simulink model "Rotorsimulation_Param_2019b"  (Simulink 10.0)
settings: Solver=ode3  StartTime=0.0  StopTime=1000  FixedStep=0.01  RelTol=1e-3  EnableMultiTasking=on
PostLoadFcn:
  | initRotorsimulation;
values from neighbouring files (symbols this model uses):
  BEMTPitchMax_deg = -30.0    [DD_Mdl.sldd]    (also in initRotorsimulationNREL5MW.m = -30)
  BladeLength_m = 61.5    [DD_Mdl.sldd]    (also in initRotorsimulationNREL5MW.m)
  BladeMass_kg = 17740.0    [DD_Mdl.sldd]    (also in initRotorsimulationNREL5MW.m = 17740)
  BladePitchMax_deg = 0.0    [DD_Mdl.sldd]    (also in initRotorsimulationNREL5MW.m = 0)
  BladePitchrateNorm_degpers = 3.0    [DD_Mdl.sldd]    (also in initRotorsimulationNREL5MW.m = 3)
  BladePitchrateStop_degpers = 9.0    [DD_Mdl.sldd]    (also in initRotorsimulationNREL5MW.m = 9)
  BladePitchStart_deg = -85.0    [DD_Mdl.sldd]    (also in initRotorsimulationNREL5MW.m = -85)
  BladePrecone_deg = 2.5    [DD_Mdl.sldd]    (also in initRotorsimulationNREL5MW.m)
  BladeTwist_deg = 13.308 13.308 13.308 13.308 13.308 13.308 13.308 13.308 13.308 13.308 13.308 13.308 13.181 12.848 12.192 11.561 11.072 10.792 10.232 9.672 9.11 8.534 7.932 7.321 6.711 6.122 5.546 4.971 4.401 3.834 3.332 2.89 2.503 2.116 1.73 1.342 0.954 0.76 0.574 0.404 0.319 0.253 0.216 0.178 0.14 0.101 0.062 0.023 0.0    [DD_Mdl.sldd]    (also in initRotorsimulationNREL5MW.m = [13.308 13.308 13.308 13.308 13.308 13.308 13.308 13.308 13.)
  cperR = 0.054 0.054 0.056 0.058 0.06 0.061 0.063 0.065 0.067 0.069 0.07 0.072 0.073 0.073 0.073 0.074 0.073 0.072 0.071 0.069 0.068 0.066 0.064 0.062 0.06 0.058 0.056 0.054 0.052 0.05 0.049 0.047 0.045 0.043 0.041 0.039 0.037 0.036 0.035 0.033 0.032 0.03 0.028 0.026 0.024 0.022 0.02 0.018 0.017    [DD_Mdl.sldd]    (also in initRotorsimulationNREL5MW.m = [0.054 0.054 0.056 0.058 0.060 0.061 0.063 0.065 0.067 0.069)
  Cut_OffWindSpeed_mpers = 25.0    [DD_Mdl.sldd]    (also in initRotorsimulationNREL5MW.m = 25)
  DownwashCorrection = 0.26    [DD_Mdl.sldd]    (also in initRotorsimulationNREL5MW.m)
  DownwashModelSwitch = 3.0    [DD_Mdl.sldd]    (also in initRotorsimulationNREL5MW.m = 3)
  drperR = 0.024 0.003 0.016 0.016 0.016 0.016 0.016 0.016 0.016 0.016 0.016 0.016 0.016 0.016 0.016 0.016 0.016 0.016 0.032 0.032 0.032 0.032 0.032 0.032 0.032 0.032 0.032 0.032 0.032 0.032 0.032 0.032 0.032 0.032 0.032 0.032 0.032 0.016 0.016 0.016 0.008 0.008 0.008 0.008 0.008 0.008 0.008 0.008 0.005    [DD_Mdl.sldd]    (also in initRotorsimulationNREL5MW.m = [0.024 0.003 0.016 0.016 0.016 0.016 0.016 0.016 0.016 0.016)
  DT_s = 0.008    [DD_Mdl.sldd]    (also in initRotorsimulationNREL5MW.m = 0.01)
  g_mpers_2 = 9.81    [DD_Mdl.sldd]    (also in initRotorsimulationNREL5MW.m)
  GeneratorEfficiency = 0.944    [DD_Mdl.sldd]    (also in initRotorsimulationNREL5MW.m)
  GeneratorOptimalModeGain_Nmper_radpers2 = 2128600    [initRotorsimulationNREL5MW.m]
  HubRadius_m = 1.5    [DD_Mdl.sldd]    (also in initRotorsimulationNREL5MW.m)
  Ki = 0.3    [initRotorsimulationNREL5MW.m]
  Kp = 0.1    [initRotorsimulationNREL5MW.m]
  mpermBl = 0.058 0.008 0.044 0.043 0.042 0.034 0.026 0.024 0.023 0.022 0.023 0.024 0.024 0.023 0.022 0.02 0.02 0.02 0.039 0.038 0.037 0.036 0.034 0.033 0.03 0.029 0.028 0.025 0.023 0.021 0.019 0.018 0.016 0.015 0.012 0.011 0.01 0.005 0.004 0.004 0.002 0.002 0.002 0.002 0.001 0.001 0.001 0.0 0.0    [DD_Mdl.sldd]    (also in initRotorsimulationNREL5MW.m = [0.058 0.008 0.044 0.043 0.042 0.034 0.026 0.024 0.023 0.022)
  nBl = 3.0    [DD_Mdl.sldd]    (also in initRotorsimulationNREL5MW.m = 3)
  nR = 49.0    [DD_Mdl.sldd]    (also in initRotorsimulationNREL5MW.m = length(drperR))
  Overhang_m = 5.0    [DD_Mdl.sldd]    (also in initRotorsimulationNREL5MW.m = 5)
  RatedOmega_RPM = 12.1    [DD_Mdl.sldd]    (also in initRotorsimulationNREL5MW.m)
  RatedWindSpeed_mpers = 11.4    [DD_Mdl.sldd]    (also in initRotorsimulationNREL5MW.m)
  rho_kgperm3 = 1.225    [DD_Mdl.sldd]    (also in initRotorsimulationNREL5MW.m)
  rperR = 0.024 0.027 0.043 0.059 0.075 0.09 0.106 0.122 0.138 0.154 0.17 0.186 0.202 0.217 0.233 0.249 0.265 0.281 0.313 0.344 0.376 0.408 0.44 0.471 0.503 0.535 0.567 0.598 0.63 0.662 0.694 0.725 0.757 0.789 0.821 0.852 0.884 0.9 0.916 0.932 0.94 0.948 0.956 0.963 0.971 0.979 0.987 0.995 1.0    [DD_Mdl.sldd]    (also in initRotorsimulationNREL5MW.m = [0.024 0.027 0.043 0.059 0.075 0.090 0.106 0.122 0.138 0.154)
  Shafttilt_deg = 5.0    [DD_Mdl.sldd]    (also in initRotorsimulationNREL5MW.m = 5)
  TipSpeedLoss = 0.0    [DD_Mdl.sldd]    (also in initRotorsimulationNREL5MW.m = 0)
  TowerDamOnperoff = 0.0    [DD_Mdl.sldd]    (also in initRotorsimulationNREL5MW.m = 0)
  TowerDragCoefficient = 0.35    [DD_Mdl.sldd]    (also in initRotorsimulationNREL5MW.m)
  TowerRadius_m = 1.935    [DD_Mdl.sldd]    (also in initRotorsimulationNREL5MW.m)
libraries: simulink x7
(part 1 of 2)
settings Model: Creator=rbartels  LastModifiedBy=ditt_aj
settings DataIOCC: LimitDataPoints=on  SignalLoggingSaveFormat=ModelDataLogs
settings OptimizationCC: ExpressionDepthLimit=2147483647  InitFltsAndDblsToZero=on
settings DebuggingCC: SolverPrmCheckMsg=warning  FcnCallInpInsideContextMsg=warning  StateNameClashWarn=warning
settings SFSimCC: SimUseLocalCustomCode=on
settings RTWCC: RTWUseLocalCustomCode=on

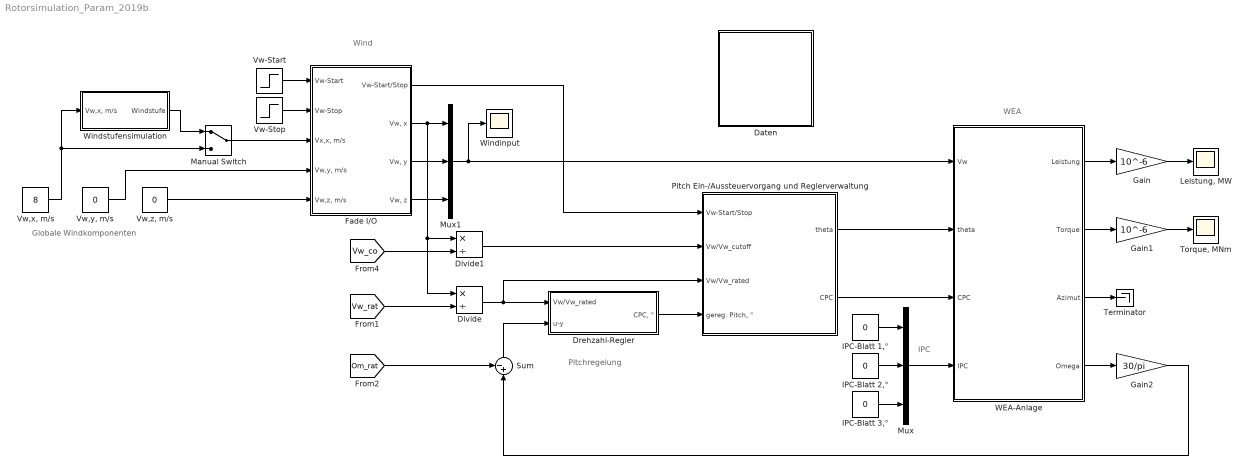
== system Rotorsimulation_Param_2019b ==
  note: Wind
  note: Pitchregelung
  note: IPC
  note: WEA
  note: Globale Windkomponenten
  Daten : Subsystem
  Divide : Product  Inputs=*/
  Divide1 : Product  Inputs=*/
  Drehzahl-Regler : Subsystem
  Fade I/O : Subsystem
  Gain : Gain  Gain=10^-6
  Gain1 : Gain  Gain=10^-6
  Gain2 : Gain  Gain=30/pi
  IPC-Blatt 1,° : Constant  Value=0
  IPC-Blatt 2,° : Constant  Value=0
  IPC-Blatt 3,° : Constant  Value=0
  "Leistung, MW" : Scope
  Manual Switch : ManualSwitch
  Mux : Mux  Inputs=3
  Mux1 : Mux  Inputs=3
  Pitch Ein-/Aussteuervorgang und Reglerverwaltung : Subsystem
  Sum : Sum  Inputs=-+|
  Terminator : Terminator
  "Torque, MNm" : Scope
  "Vw,x, m/s " : Constant  Value=8
  "Vw,y, m/s" : Constant  Value=0
  "Vw,z, m/s" : Constant  Value=0
  Vw-Start : Step  SampleTime=0
  Vw-Stop : Step  Time=2000  Before=1  After=0  SampleTime=0
  WEA-Anlage : Subsystem
  Windinput : Scope
  Windstufensimulation : Subsystem
  wires:
  Fade I/O/2("Vw, x") -> Mux1/1, Divide/1, Divide1/1
  Vw-Start/1 -> Fade I/O/1(Vw-Start)
  Vw-Stop/1 -> Fade I/O/2(Vw-Stop)
  WEA-Anlage/1(Leistung) -> Gain/1
  "Vw,y, m/s"/1 -> Fade I/O/4("Vw,y, m/s")
  "Vw,z, m/s"/1 -> Fade I/O/5("Vw,z, m/s")
  Fade I/O/4("Vw, z") -> Mux1/3
  Fade I/O/3("Vw, y") -> Mux1/2
  WEA-Anlage/2(Torque) -> Gain1/1
  Gain/1 -> "Leistung, MW"/1
  Gain1/1 -> "Torque, MNm"/1
  IPC-Blatt 3,°/1 -> Mux/3
  WEA-Anlage/3(Azimut) -> Terminator/1
  WEA-Anlage/4(Omega) -> Gain2/1
  Sum/1 -> Drehzahl-Regler/2(u-y)
  Drehzahl-Regler/1("CPC, °") -> Pitch Ein-/Aussteuervorgang und Reglerverwaltung/4("gereg. Pitch, °")
  [Vw_rat] -> Divide/2
  Divide/1 -> Drehzahl-Regler/1(Vw/Vw_rated), Pitch Ein-/Aussteuervorgang und Reglerverwaltung/3(Vw/Vw_rated)
  [Om_rat] -> Sum/1
  Gain2/1 -> Sum/2
  Mux1/1 -> WEA-Anlage/1(Vw), Windinput/1
  Fade I/O/1(Vw-Start/Stop) -> Pitch Ein-/Aussteuervorgang und Reglerverwaltung/1(Vw-Start/Stop)
  Manual Switch/1 -> Fade I/O/3("Vx,x, m/s")
  "Vw,x, m/s "/1 -> Windstufensimulation/1("Vw,x, m/s"), Manual Switch/2
  Windstufensimulation/1(" Windstufe") -> Manual Switch/1
  Divide1/1 -> Pitch Ein-/Aussteuervorgang und Reglerverwaltung/2(Vw/Vw_cutoff)
  [Vw_co] -> Divide1/2
  IPC-Blatt 2,°/1 -> Mux/2
  IPC-Blatt 1,°/1 -> Mux/1
  Mux/1 -> WEA-Anlage/4(IPC)
  Pitch Ein-/Aussteuervorgang und Reglerverwaltung/2(CPC) -> WEA-Anlage/3(CPC)
  Pitch Ein-/Aussteuervorgang und Reglerverwaltung/1(theta) -> WEA-Anlage/2(theta)

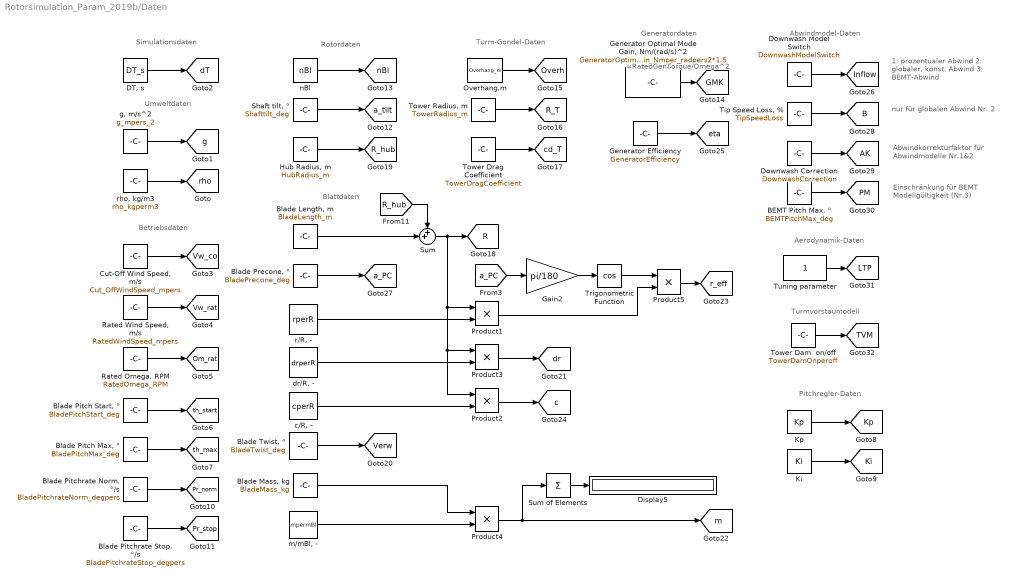
== system Rotorsimulation_Param_2019b/Daten ==
  note: Simulationsdaten
  note: Umweltdaten
  note: Betriebsdaten
  note: Pitchregler-Daten
  note: =RatedGenTorque/Omega^2
  note: Rotordaten
  note: Turm-Gondel-Daten
  note: Generatordaten
  note: Blattdaten
  note: 1: prozentualer Abwind
      | 2: globaler, konst. Abwind
      | 3: BEMT-Abwind
  note: Abwindmodel-Daten
  note: nur für globalen Abwind Nr. 2
  note: Abwindkorrekturfaktor für
      | Abwindmodelle Nr.1&2
  note: Einschränkung für BEMT
      | Modellgültigkeit (Nr.3)
  note: Aerodynamik-Daten
  note: Turmvorstaumodell
  "BEMT Pitch Max, °" : Constant  Value=BEMTPitchMax_deg
  "Blade Length, m" : Constant  Value=BladeLength_m
  "Blade Mass, kg" : Constant  Value=BladeMass_kg
  "Blade Pitch Max, °" : Constant  Value=BladePitchMax_deg
  "Blade Pitch Start, °" : Constant  Value=BladePitchStart_deg
  Blade Pitchrate Norm. °/s : Constant  Value=BladePitchrateNorm_degpers
  Blade Pitchrate Stop. °/s : Constant  Value=BladePitchrateStop_degpers
  "Blade Precone, °" : Constant  Value=BladePrecone_deg
  "Blade Twist, °" : Constant  Value=BladeTwist_deg
  "Cut-Off Wind Speed, m/s" : Constant  Value=Cut_OffWindSpeed_mpers
  "DT, s" : Constant  Value=DT_s
  Display5 : Display
  Downwash Correction : Constant  Value=DownwashCorrection
  Downwash Model Switch : Constant  Value=DownwashModelSwitch
  Gain2 : Gain  Gain=pi/180
  Generator Efficiency : Constant  Value=GeneratorEfficiency
  "Generator Optimal Mode Gain, Nm/(rad/s)^2" : Constant  Value=GeneratorOptimalModeGain_Nmper_radpers2*1.5
  "Hub Radius, m" : Constant  Value=HubRadius_m
  Ki : Constant  Value=Ki
  Kp : Constant  Value=Kp
  Overhang,m : Constant  Value=Overhang_m
  Product{1..5} (5 alike) : Product  RndMeth=Zero
  "Rated Omega, RPM" : Constant  Value=RatedOmega_RPM
  "Rated Wind Speed, m/s" : Constant  Value=RatedWindSpeed_mpers
  "Shaft tilt, °" : Constant  Value=Shafttilt_deg
  Sum : Sum  Inputs=++|
  Sum of Elements : Sum  Inputs=+
  "Tip Speed Loss, %" : Constant  Value=TipSpeedLoss
  Tower Dam  on/off : Constant  Value=TowerDamOnperoff
  Tower Drag Coefficient : Constant  Value=TowerDragCoefficient
  "Tower Radius, m" : Constant  Value=TowerRadius_m
  Trigonometric Function : Trigonometry  Operator=cos
  Tuning parameter : Constant
  "c/R, -" : Constant  Value=cperR
  "dr/R, -" : Constant  Value=drperR
  "g, m/s^2" : Constant  Value=g_mpers_2
  "m/mBl, - " : Constant  Value=mpermBl
  nBl : Constant  Value=nBl
  "r/R, -" : Constant  Value=rperR
  "rho, kg/m3" : Constant  Value=rho_kgperm3
  tag scope: AK=global, B=global, GMK=global, Inflow=global, Ki=global, Kp=global, LTP=global, Om_rat=global, Overh=global, PM=global, Pr_norm=global, Pr_stop=global, R=global, R_T=global, R_hub=global, TVM=global, Verw=global, Vw_co=global, Vw_rat=global, a_PC=global, a_tilt=global, c=global, cd_T=global, dT=global, dr=global, eta=global, g=global, m=global, nBl=global, r_eff=global, rho=global, th_max=global, th_start=global
  wires:
  "rho, kg/m3"/1 -> [rho]
  "g, m/s^2"/1 -> [g]
  "DT, s"/1 -> [dT]
  "Cut-Off Wind Speed, m/s"/1 -> [Vw_co]
  "Rated Wind Speed, m/s"/1 -> [Vw_rat]
  "Rated Omega, RPM"/1 -> [Om_rat]
  "Blade Pitch Start, °"/1 -> [th_start]
  "Blade Pitch Max, °"/1 -> [th_max]
  Ki/1 -> [Ki]
  Kp/1 -> [Kp]
  Blade Pitchrate Norm. °/s/1 -> [Pr_norm]
  Blade Pitchrate Stop. °/s/1 -> [Pr_stop]
  nBl/1 -> [nBl]
  "Generator Optimal Mode Gain, Nm/(rad/s)^2"/1 -> [GMK]
  "Shaft tilt, °"/1 -> [a_tilt]
  Overhang,m/1 -> [Overh]
  "Tower Radius, m"/1 -> [R_T]
  Tower Drag Coefficient/1 -> [cd_T]
  "r/R, -"/1 -> Product1/2
  "c/R, -"/1 -> Product2/2
  "Blade Twist, °"/1 -> [Verw]
  "m/mBl, - "/1 -> Product4/2
  "dr/R, -"/1 -> Product3/2
  Sum of Elements/1 -> Display5/1
  Gain2/1 -> Trigonometric Function/1
  Trigonometric Function/1 -> Product5/1
  Product5/1 -> [r_eff]
  Product1/1 -> Product5/2
  Product3/1 -> [dr]
  Product2/1 -> [c]
  Product4/1 -> [m], Sum of Elements/1
  "Hub Radius, m"/1 -> [R_hub]
  Sum/1 -> [R], Product1/1, Product3/1, Product2/1
  "Blade Length, m"/1 -> Sum/2
  [R_hub] -> Sum/1
  "Blade Mass, kg"/1 -> Product4/1
  "Blade Precone, °"/1 -> [a_PC]
  [a_PC] -> Gain2/1
  Generator Efficiency/1 -> [eta]
  Downwash Model Switch/1 -> [Inflow]
  "Tip Speed Loss, %"/1 -> [B]
  Downwash Correction/1 -> [AK]
  "BEMT Pitch Max, °"/1 -> [PM]
  Tuning parameter/1 -> [LTP]
  Tower Dam  on/off/1 -> [TVM]

== system Rotorsimulation_Param_2019b/Drehzahl-Regler ==
  Vw/Vw_rated : Inport
  u-y : Inport  Port=2
  Diff : Constant  Value=0
  Gain3 : Gain  Gain=180/pi
  PI-Regler : Subsystem
  Saturation Dynamic : simulink/Discontinuities/Saturation Dynamic  OutMin=[]  OutMax=[]  OutDataTypeStr=Inherit: Same as second input  OutDataType=sfix(16)  OutScaling=2^-10  DoSatur=off
  Switch : Switch  Criteria=u2 > Threshold  Threshold=1
  Verstärkungen : Subsystem
  "CPC, °" : Outport  VectorParamsAs1DForOutWhenUnconnected=off
  wires:
  PI-Regler/1(e) -> Gain3/1
  Verstärkungen/1(Verstärkungen) -> PI-Regler/2(Verstärkungen)
  Gain3/1 -> Saturation Dynamic/2
  Saturation Dynamic/1 -> "CPC, °"/1
  [th_max] -> Saturation Dynamic/1
  [th_start] -> Saturation Dynamic/3
  Diff/1 -> Switch/3
  u-y/1 -> Switch/1  "diff"
  Vw/Vw_rated/1 -> Switch/2
  Switch/1 -> PI-Regler/1(u-y)

== system Rotorsimulation_Param_2019b/Fade I/O ==
  Vw-Start : Inport
  Vw-Stop : Inport  Port=2
  "Vx,x, m/s" : Inport  Port=3
  "Vw,y, m/s" : Inport  Port=4
  "Vw,z, m/s" : Inport  Port=5
  Demux : Demux  Outputs=3
  Mux2 : Mux  Inputs=3
  Product : Product  RndMeth=Zero
  Product1 : Product  RndMeth=Zero
  Rate Limiter1 : RateLimiter  SampleTimeMode=inherited
  Vw-Start/Stop : Outport  VectorParamsAs1DForOutWhenUnconnected=off
  "Vw, x" : Outport  Port=2  VectorParamsAs1DForOutWhenUnconnected=off
  "Vw, y" : Outport  Port=3  VectorParamsAs1DForOutWhenUnconnected=off
  "Vw, z" : Outport  Port=4  VectorParamsAs1DForOutWhenUnconnected=off
  tag scope: Vw_in=global
  wires:
  Product1/1 -> Rate Limiter1/1
  Rate Limiter1/1 -> Demux/1
  "Vx,x, m/s"/1 -> Mux2/1
  "Vw,y, m/s"/1 -> Mux2/2
  "Vw,z, m/s"/1 -> Mux2/3
  Mux2/1 -> Product1/2
  Demux/1 -> "Vw, x"/1, [Vw_in]
  Demux/3 -> "Vw, z"/1
  Demux/2 -> "Vw, y"/1
  Vw-Start/1 -> Product/1
  Vw-Stop/1 -> Product/2
  Product/1 -> Product1/1, Vw-Start/Stop/1

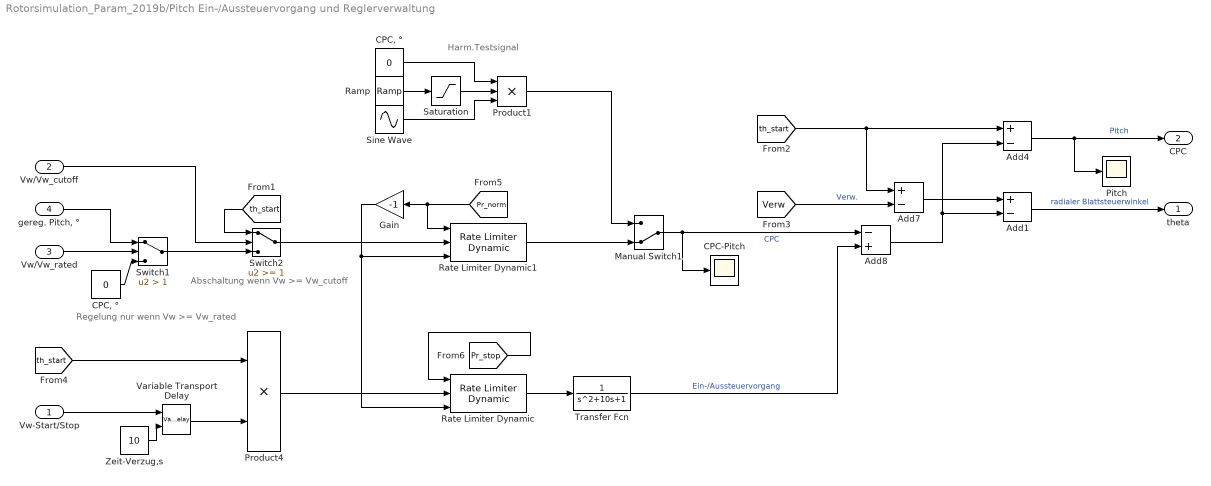
== system Rotorsimulation_Param_2019b/Pitch Ein-/Aussteuervorgang und Reglerverwaltung ==
  note: Harm.Testsignal
  note: Regelung nur wenn Vw >= Vw_rated
  note: Abschaltung wenn Vw >= Vw_cutoff
  Vw-Start/Stop : Inport
  Vw/Vw_cutoff : Inport  Port=2
  Vw/Vw_rated : Inport  Port=3
  "gereg. Pitch, °" : Inport  Port=4
  " CPC, ° " : Constant  Value=0
  " Pitch " : Scope
  Add1 : Sum  Inputs=+-
  Add4 : Sum  Inputs=+-
  Add7 : Sum  Inputs=+-
  Add8 : Sum  Inputs=-+
  "CPC, °" : Constant  Value=0
  CPC-Pitch : Scope
  Gain : Gain  Gain=-1
  Manual Switch1 : ManualSwitch  CurrentSetting=0
  Product1 : Product  Inputs=3  RndMeth=Zero
  Product4 : Product  RndMeth=Zero
  Ramp : simulink/Sources/Ramp  slope=0.1  start=200  InitialOutput=0
  Rate Limiter Dynamic : simulink/Discontinuities/Rate Limiter Dynamic
      settings: SourceProductName=Simulink
  Rate Limiter Dynamic1 : simulink/Discontinuities/Rate Limiter Dynamic
      settings: SourceProductName=Simulink
  Saturation : Saturate  UpperLimit=1  LowerLimit=0
  Sine Wave : Sin  Frequency=0.1  SampleTime=0
  Switch1 : Switch  Criteria=u2 > Threshold  Threshold=1
  Switch2 : Switch  Threshold=1
  Transfer Fcn : TransferFcn  Denominator=[1 10 1]
  Variable Transport Delay : VariableTransportDelay  VariableDelayType=Variable transport delay  MaximumDelay=10
  Zeit-Verzug,s : Constant  Value=10
  theta : Outport  VectorParamsAs1DForOutWhenUnconnected=off
  CPC : Outport  Port=2  VectorParamsAs1DForOutWhenUnconnected=off
  wires:
  Rate Limiter Dynamic/1 -> Transfer Fcn/1
  Product4/1 -> Rate Limiter Dynamic/2
  [th_start] -> Product4/1
  Transfer Fcn/1 -> Add8/2  "Ein-/Aussteuervorgang"
  Variable Transport Delay/1 -> Product4/2
  Vw-Start/Stop/1 -> Variable Transport Delay/1
  Zeit-Verzug,s/1 -> Variable Transport Delay/2
  [Pr_stop] -> Rate Limiter Dynamic/1
  Ramp/1 -> Saturation/1
  Sine Wave/1 -> Product1/3
  Saturation/1 -> Product1/2
  Product1/1 -> Manual Switch1/1
  " CPC, ° "/1 -> Switch1/3
  "CPC, °"/1 -> Product1/1
  Manual Switch1/1 -> Add8/1, CPC-Pitch/1  "CPC"
  Switch1/1 -> Switch2/3
  Switch2/1 -> Rate Limiter Dynamic1/2
  [th_start] -> Switch2/1
  Vw/Vw_cutoff/1 -> Switch2/2
  Vw/Vw_rated/1 -> Switch1/2
  "gereg. Pitch, °"/1 -> Switch1/1
  [th_start] -> Add4/1, Add7/1
  Add7/1 -> Add1/1
  [Verw] -> Add7/2  "Verw."
  Add4/1 -> " Pitch "/1, CPC/1  "Pitch"
  Add8/1 -> Add4/2, Add1/2
  Add1/1 -> theta/1  "radialer Blattsteuerwinkel"
  Rate Limiter Dynamic1/1 -> Manual Switch1/2
  [Pr_norm] -> Rate Limiter Dynamic1/1, Gain/1
  Gain/1 -> Rate Limiter Dynamic1/3, Rate Limiter Dynamic/3

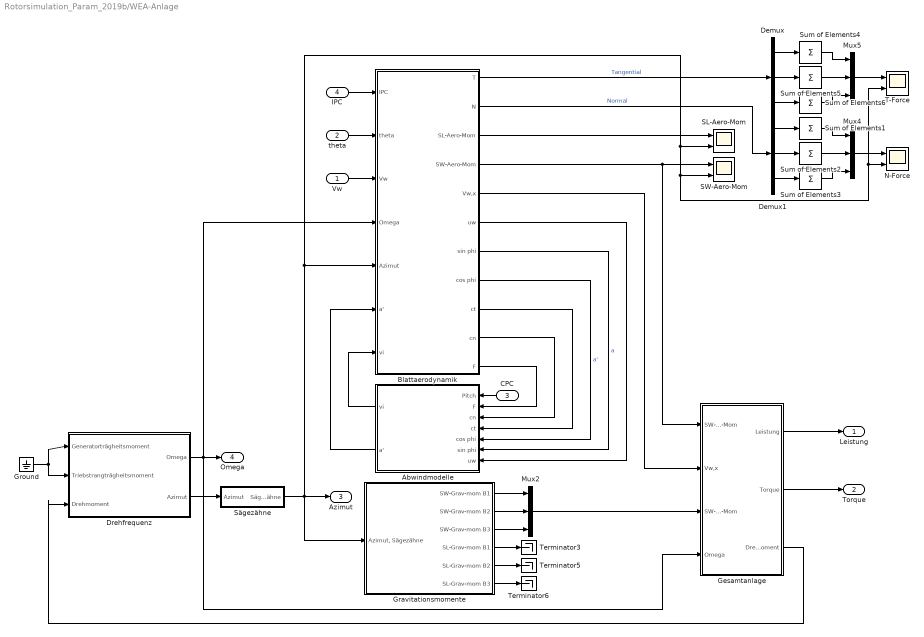
== system Rotorsimulation_Param_2019b/WEA-Anlage ==
  Vw : Inport
  theta : Inport  Port=2
  CPC : Inport  Port=3
  IPC : Inport  Port=4
  Abwindmodelle : Subsystem
  Blattaerodynamik : Subsystem
  Demux : Demux  Outputs=3
  Demux1 : Demux  Outputs=3
  Drehfrequenz : Subsystem
  Gesamtanlage : Subsystem
  Gravitationsmomente : Subsystem
  Ground : Ground
  Mux2 : Mux  Inputs=3
  Mux4 : Mux  Inputs=3
  Mux5 : Mux  Inputs=3
  N-Force : Scope  NumInputPorts=2
  SL-Aero-Mom : Scope  NumInputPorts=2
  SW-Aero-Mom : Scope  NumInputPorts=2
  Sum of Elements{1..6} (6 alike) : Sum  Inputs=+
  Sägezähne : Subsystem
  T-Force : Scope  NumInputPorts=2
  Terminator3 : Terminator
  Terminator5 : Terminator
  Terminator6 : Terminator
  Leistung : Outport  VectorParamsAs1DForOutWhenUnconnected=off
  Torque : Outport  Port=2  VectorParamsAs1DForOutWhenUnconnected=off
  Azimut : Outport  Port=3  VectorParamsAs1DForOutWhenUnconnected=off
  Omega : Outport  Port=4  VectorParamsAs1DForOutWhenUnconnected=off
  wires:
  Blattaerodynamik/1(T) -> Demux/1  "Tangential"
  Blattaerodynamik/2(N) -> Demux1/1  "Normal"
  Sägezähne/1(Sägezähne) -> Gravitationsmomente/1("Azimut, Sägezähne"), Blattaerodynamik/5(Azimut), SL-Aero-Mom/2, SW-Aero-Mom/2, N-Force/2, T-Force/2, Azimut/1
  Drehfrequenz/2(Azimut) -> Sägezähne/1(Azimut)
  Blattaerodynamik/4(SW-Aero-Mom) -> Gesamtanlage/1(SW-Aero-Mom), SW-Aero-Mom/1
  Blattaerodynamik/3(SL-Aero-Mom) -> SL-Aero-Mom/1
  Gravitationsmomente/1(SW-Grav-mom B1) -> Mux2/1
  Gravitationsmomente/2(SW-Grav-mom B2) -> Mux2/2
  Gravitationsmomente/3(SW-Grav-mom B3) -> Mux2/3
  Gesamtanlage/2(Torque) -> Torque/1
  Abwindmodelle/1(vi) -> Blattaerodynamik/7(vi)
  Blattaerodynamik/8(cos phi) -> Abwindmodelle/5(cos phi)  "a'"
  Blattaerodynamik/7(sin phi) -> Abwindmodelle/6(sin phi)  "a"
  Blattaerodynamik/10(cn) -> Abwindmodelle/3(cn)
  Blattaerodynamik/9(ct) -> Abwindmodelle/4(ct)
  Abwindmodelle/2(a') -> Blattaerodynamik/6(a')
  theta/1 -> Blattaerodynamik/2(theta)
  Blattaerodynamik/11(F) -> Abwindmodelle/2(F)
  Gravitationsmomente/4(SL-Grav-mom B1) -> Terminator3/1
  Gravitationsmomente/6(SL-Grav-mom B3) -> Terminator6/1
  Gravitationsmomente/5(SL-Grav-mom B2) -> Terminator5/1
  Vw/1 -> Blattaerodynamik/3(Vw)
  Drehfrequenz/1(Omega) -> Gesamtanlage/4(Omega), Omega/1, Blattaerodynamik/4(Omega)
  Mux2/1 -> Gesamtanlage/3(SW-Grav-Mom)
  Gesamtanlage/1(Leistung) -> Leistung/1
  Gesamtanlage/3(Drehmoment) -> Drehfrequenz/3(Drehmoment)
  Demux1/1 -> Sum of Elements1/1
  Demux1/2 -> Sum of Elements2/1
  Demux1/3 -> Sum of Elements3/1
  Sum of Elements1/1 -> Mux4/1
  Sum of Elements2/1 -> Mux4/2
  Mux4/1 -> N-Force/1
  Demux/1 -> Sum of Elements4/1
  Demux/2 -> Sum of Elements5/1
  Demux/3 -> Sum of Elements6/1
  Sum of Elements4/1 -> Mux5/1
  Sum of Elements6/1 -> Mux5/3
  Sum of Elements5/1 -> Mux5/2
  Mux5/1 -> T-Force/1
  Blattaerodynamik/5(Vw,x) -> Gesamtanlage/2(Vw,x)
  Blattaerodynamik/6(" uw") -> Abwindmodelle/7(uw)
  IPC/1 -> Blattaerodynamik/1(IPC)
  CPC/1 -> Abwindmodelle/1(Pitch)
  Ground/1 -> Drehfrequenz/1(Generatorträgheitsmoment), Drehfrequenz/2(Triebstrangträgheitsmoment)
  Sum of Elements3/1 -> Mux4/3

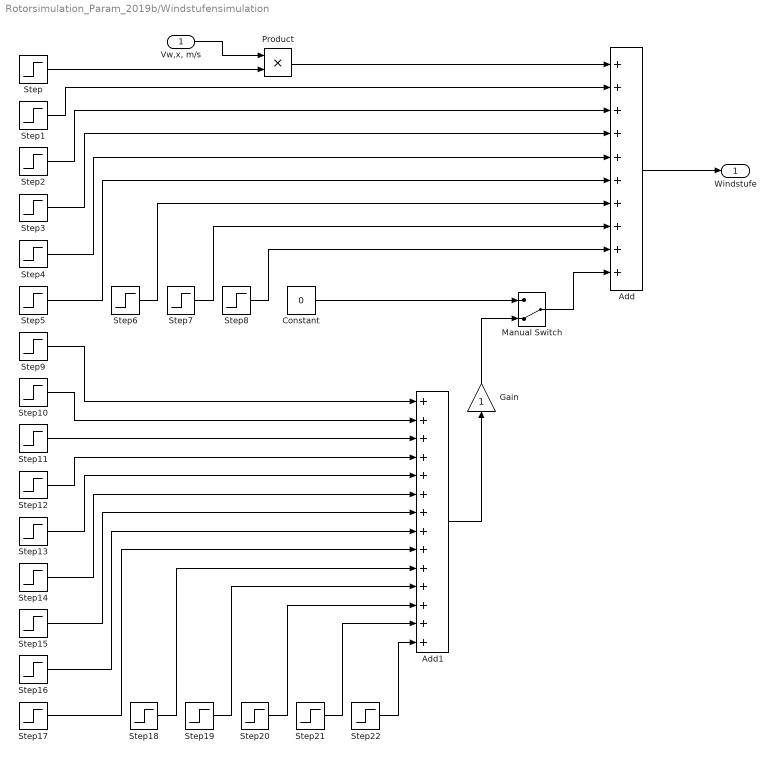
== system Rotorsimulation_Param_2019b/Windstufensimulation ==
  "Vw,x, m/s" : Inport
  Add : Sum  Inputs=++++++++++
  Add1 : Sum  Inputs=++++++++++++++
  Constant : Constant  Value=0
  Gain : Gain
  Manual Switch : ManualSwitch  CurrentSetting=0
  Product : Product  RndMeth=Zero
  Step : Step  SampleTime=0
  Step1 : Step  Time=50  SampleTime=0
  Step10 : Step  Time=500  SampleTime=0
  Step11 : Step  Time=550  SampleTime=0
  Step12 : Step  Time=600  SampleTime=0
  Step13 : Step  Time=650  SampleTime=0
  Step14 : Step  Time=700  SampleTime=0
  Step15 : Step  Time=750  SampleTime=0
  Step16 : Step  Time=800  SampleTime=0
  Step17 : Step  Time=850  SampleTime=0
  Step18 : Step  Time=900  SampleTime=0
  Step19 : Step  Time=950  SampleTime=0
  Step2 : Step  Time=100  SampleTime=0
  Step20 : Step  Time=1000  SampleTime=0
  Step21 : Step  Time=1050  SampleTime=0
  Step22 : Step  Time=1100  SampleTime=0
  Step3 : Step  Time=150  SampleTime=0
  Step4 : Step  Time=200  SampleTime=0
  Step5 : Step  Time=250  SampleTime=0
  Step6 : Step  Time=300  SampleTime=0
  Step7 : Step  Time=350  SampleTime=0
  Step8 : Step  Time=400  SampleTime=0
  Step9 : Step  Time=450  SampleTime=0
  " Windstufe" : Outport  VectorParamsAs1DForOutWhenUnconnected=off
  wires:
  Step8/1 -> Add/9
  Step7/1 -> Add/8
  Step6/1 -> Add/7
  Step5/1 -> Add/6
  Step4/1 -> Add/5
  Step3/1 -> Add/4
  Step2/1 -> Add/3
  Step1/1 -> Add/2
  Step/1 -> Product/2
  Product/1 -> Add/1
  "Vw,x, m/s"/1 -> Product/1
  Add/1 -> " Windstufe"/1
  Step20/1 -> Add1/12
  Step19/1 -> Add1/11
  Step11/1 -> Add1/3
  Add1/1 -> Gain/1
  Step10/1 -> Add1/2
  Step9/1 -> Add1/1
  Step12/1 -> Add1/4
  Step13/1 -> Add1/5
  Step14/1 -> Add1/6
  Step15/1 -> Add1/7
  Step16/1 -> Add1/8
  Step17/1 -> Add1/9
  Step18/1 -> Add1/10
  Step21/1 -> Add1/13
  Step22/1 -> Add1/14
  Constant/1 -> Manual Switch/1
  Manual Switch/1 -> Add/10
  Gain/1 -> Manual Switch/2

== system Rotorsimulation_Param_2019b/Drehzahl-Regler/PI-Regler ==
  u-y : Inport
  Verstärkungen : Inport  Port=2
  Demux : Demux  Outputs=3
  Diskreter Integrierer : Subsystem
  Product : Product  RndMeth=Zero
  Product1 : Product  RndMeth=Zero
  Product2 : Product  RndMeth=Zero
  Sum : Sum  Inputs=++|  SaturateOnIntegerOverflow=on  InputSameDT=on  OutDataTypeStr=Inherit: Same as first input
  e : Outport  VectorParamsAs1DForOutWhenUnconnected=off
  wires:
  Demux/1 -> Product/2
  Verstärkungen/1 -> Demux/1
  Demux/2 -> Product1/2
  Product/1 -> Sum/1
  Diskreter Integrierer/1(Out1) -> Sum/2
  Product1/1 -> Diskreter Integrierer/1(In1)
  Sum/1 -> Product2/1
  u-y/1 -> Product/1, Product1/1
  Product2/1 -> e/1
  Demux/3 -> Product2/2

== system Rotorsimulation_Param_2019b/Drehzahl-Regler/Verstärkungen ==
  note: PI-Regler
  Gain7 : Gain  Gain=-1
  Khub : Constant
  Mux9 : Mux  Inputs=3
  Verstärkungen : Outport  VectorParamsAs1DForOutWhenUnconnected=off
  wires:
  Gain7/1 -> Mux9/3
  Khub/1 -> Gain7/1
  [Ki] -> Mux9/2
  [Kp] -> Mux9/1
  Mux9/1 -> Verstärkungen/1

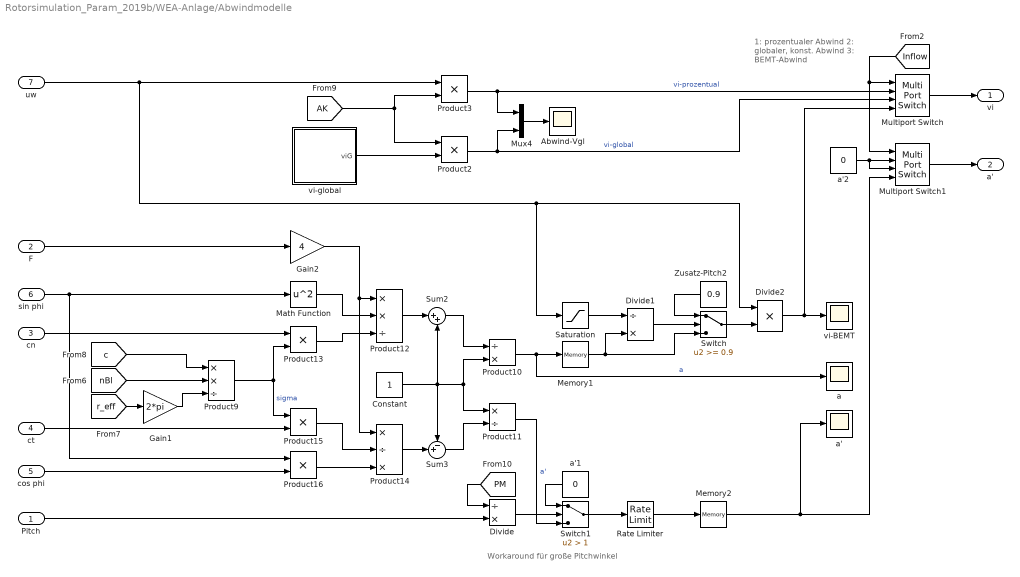
== system Rotorsimulation_Param_2019b/WEA-Anlage/Abwindmodelle ==
  note: Workaround für große Pitchwinkel
  note: 1: prozentualer Abwind
      | 2: globaler, konst. Abwind
      | 3: BEMT-Abwind
  Pitch : Inport
  F : Inport  Port=2
  cn : Inport  Port=3
  ct : Inport  Port=4
  cos phi : Inport  Port=5
  sin phi : Inport  Port=6
  uw : Inport  Port=7
  " a " : Scope
  " a' " : Scope
  Abwind-Vgl : Scope
  Constant : Constant
  Divide : Product  Inputs=/*
  Divide1 : Product  Inputs=/*
  Divide2 : Product
  Gain1 : Gain  Gain=2*pi
  Gain2 : Gain  Gain=4
  Math Function : Math  Operator=square  SaturateOnIntegerOverflow=on
  Memory1 : Memory
  Memory2 : Memory
  Multiport Switch : MultiPortSwitch  RndMeth=Nearest
  Multiport Switch1 : MultiPortSwitch  RndMeth=Nearest
  Mux4 : Mux  Inputs=2
  Product10 : Product  Inputs=/*  RndMeth=Zero
  Product11 : Product  Inputs=*/  RndMeth=Zero
  Product12 : Product  Inputs=**/  RndMeth=Zero
  Product{2..3,13,15..16} (5 alike) : Product  RndMeth=Zero
  Product14 : Product  Inputs=*/*  RndMeth=Zero
  Product9 : Product  Inputs=**/  RndMeth=Zero
  Rate Limiter : RateLimiter  SampleTimeMode=inherited
  Saturation : Saturate  UpperLimit=inf  LowerLimit=0.01
  Sum2 : Sum  Inputs=|++
  Sum3 : Sum  Inputs=-+|
  Switch : Switch  Threshold=0.9
  Switch1 : Switch  Criteria=u2 > Threshold  Threshold=1
  Zusatz-Pitch2 : Constant  Value=0.9
  a'1 : Constant  Value=0
  a'2 : Constant  Value=0
  vi-BEMT : Scope
  vi-global : Subsystem
  vi : Outport  VectorParamsAs1DForOutWhenUnconnected=off
  a' : Outport  Port=2  VectorParamsAs1DForOutWhenUnconnected=off
  wires:
  vi-global/1(viG) -> Product2/2
  Product2/1 -> Mux4/2, Multiport Switch/3  "vi-global"
  Saturation/1 -> Divide1/1
  Zusatz-Pitch2/1 -> Switch/1
  Memory1/1 -> Divide1/2, Switch/3
  Switch/1 -> Divide2/2
  Divide1/1 -> Switch/2
  Divide2/1 -> vi-BEMT/1, Multiport Switch/4
  [Inflow] -> Multiport Switch/1, Multiport Switch1/1
  Mux4/1 -> Abwind-Vgl/1
  Product3/1 -> Mux4/1, Multiport Switch/2  "vi-prozentual"
  uw/1 -> Saturation/1, Divide2/1, Product3/1
  Multiport Switch/1 -> vi/1
  cos phi/1 -> Product16/2
  sin phi/1 -> Math Function/1, Product16/1
  Constant/1 -> Sum3/1, Sum2/2, Product11/1, Product10/2
  Math Function/1 -> Product12/2
  Product13/1 -> Product12/3
  Product9/1 -> Product13/2, Product15/1  "sigma"
  cn/1 -> Product13/1
  Product16/1 -> Product14/3
  ct/1 -> Product15/2
  Product12/1 -> Sum2/1
  Product14/1 -> Sum3/2
  Sum2/1 -> Product10/1
  Sum3/1 -> Product11/2
  Product10/1 -> Memory1/1, " a "/1  "a"
  Product11/1 -> Switch1/3  "a'"
  [c] -> Product9/1
  [nBl] -> Product9/2
  [r_eff] -> Gain1/1
  Gain1/1 -> Product9/3
  a'2/1 -> Multiport Switch1/2, Multiport Switch1/3
  Multiport Switch1/1 -> a'/1
  F/1 -> Gain2/1
  Gain2/1 -> Product12/1, Product14/1
  Product15/1 -> Product14/2
  Pitch/1 -> Divide/2
  Divide/1 -> Switch1/2
  a'1/1 -> Switch1/1
  [PM] -> Divide/1
  Switch1/1 -> Rate Limiter/1
  Rate Limiter/1 -> Memory2/1
  Memory2/1 -> " a' "/1, Multiport Switch1/4
  [AK] -> Product3/2, Product2/1

== system Rotorsimulation_Param_2019b/WEA-Anlage/Blattaerodynamik ==
  IPC : Inport
  theta : Inport  Port=2
  Vw : Inport  Port=3
  Omega : Inport  Port=4
  Azimut : Inport  Port=5
  a' : Inport  Port=6
  vi : Inport  Port=7
  Anströmung : Subsystem
  Beiwerte1 : Subsystem
  Beiwerte2 : Subsystem
  Blattbiegemomente : Subsystem
  Gain5 : Gain  Gain=pi/180
  Komponenten für BEMT : Subsystem
  Normal-/Tangentialkraft : Subsystem
  Tip&Hub-Loss-Faktor : Subsystem
  T : Outport  VectorParamsAs1DForOutWhenUnconnected=off
  N : Outport  Port=2  VectorParamsAs1DForOutWhenUnconnected=off
  SL-Aero-Mom : Outport  Port=3  VectorParamsAs1DForOutWhenUnconnected=off
  SW-Aero-Mom : Outport  Port=4  VectorParamsAs1DForOutWhenUnconnected=off
  Vw,x : Outport  Port=5  VectorParamsAs1DForOutWhenUnconnected=off
  " uw" : Outport  Port=6  VectorParamsAs1DForOutWhenUnconnected=off
  sin phi : Outport  Port=7  VectorParamsAs1DForOutWhenUnconnected=off
  cos phi : Outport  Port=8  VectorParamsAs1DForOutWhenUnconnected=off
  ct : Outport  Port=9  VectorParamsAs1DForOutWhenUnconnected=off
  cn : Outport  Port=10  VectorParamsAs1DForOutWhenUnconnected=off
  F : Outport  Port=11  VectorParamsAs1DForOutWhenUnconnected=off
  wires:
  Beiwerte2/1(cl) -> Normal-/Tangentialkraft/1(cl)
  Beiwerte2/2(cd) -> Normal-/Tangentialkraft/2(cd)
  Anströmung/2(phi) -> Normal-/Tangentialkraft/3("phi, rad")
  Anströmung/3(V^2) -> Normal-/Tangentialkraft/4(V^2)
  Vw/1 -> Anströmung/3(Vw)
  Omega/1 -> Anströmung/5(Omega)
  Normal-/Tangentialkraft/1(T) -> T/1, Blattbiegemomente/1(T)
  Normal-/Tangentialkraft/2(N) -> N/1, Blattbiegemomente/2(N)
  Komponenten für BEMT/1(sin phi) -> sin phi/1, Tip&Hub-Loss-Faktor/1(sin phi)
  theta/1 -> Anströmung/2(theta)
  vi/1 -> Anströmung/4(vi)
  Komponenten für BEMT/3(ct) -> ct/1
  Komponenten für BEMT/4(cn) -> cn/1
  a'/1 -> Anströmung/6(a')
  Anströmung/1(alf_eff) -> Beiwerte2/1("alf_eff, rad")
  Tip&Hub-Loss-Faktor/1(F) -> F/1
  Azimut/1 -> Gain5/1
  Gain5/1 -> Anströmung/7(Azimut)
  Anströmung/5(uw) -> " uw"/1
  Anströmung/4(Vw,x) -> Vw,x/1
  Anströmung/6(phi BEMT) -> Komponenten für BEMT/1("phi, BEMT")
  Komponenten für BEMT/2(cos phi) -> cos phi/1
  Anströmung/7(alf_eff_BEMT) -> Beiwerte1/1("alf_eff, rad")
  Beiwerte1/1(cl) -> Komponenten für BEMT/2(cl)
  Beiwerte1/2(cd) -> Komponenten für BEMT/3(cd)
  Blattbiegemomente/1(SW-Aero-Mom) -> SW-Aero-Mom/1
  Blattbiegemomente/2(SL-Aero-Mom) -> SL-Aero-Mom/1
  IPC/1 -> Anströmung/1(IPC)

== system Rotorsimulation_Param_2019b/WEA-Anlage/Drehfrequenz ==
  note: Omega = Omega0 + dOm/dt*t
  note: Psi = Psi0 + Omega0*t + 1/2*dOm/dt*t^2
  note: Rotorträgheits-
      | moment
  Generatorträgheitsmoment : Inport
  Triebstrangträgheitsmoment : Inport  Port=2
  Drehmoment : Inport  Port=3
  Azimut1 : Scope
  Divide : Product  Inputs=*/
  Gain : Gain  Gain=1/2
  Gain4 : Gain  Gain=180/pi
  Math Function : Math  Operator=square  SaturateOnIntegerOverflow=on
  Math Function5 : Math  Operator=square  SaturateOnIntegerOverflow=on
  Memory1 : Memory
  Memory2 : Memory
  Memory5 : Memory
  Omega1 : Scope
  Product1 : Product  RndMeth=Zero
  Product2 : Product  RndMeth=Zero
  Product3 : Product  RndMeth=Zero
  Product4 : Product  Inputs=3  RndMeth=Zero
  Sum of Elements : Sum  Inputs=+
  Sum1 : Sum  Inputs=+++
  Sum2 : Sum  Inputs=++|
  Sum6 : Sum  Inputs=++|
  Sum7 : Sum  Inputs=+|+
  Trägheitsmoment : Display
      settings: Decimation=100
  Omega : Outport  VectorParamsAs1DForOutWhenUnconnected=off
  Azimut : Outport  Port=2  VectorParamsAs1DForOutWhenUnconnected=off
  wires:
  Drehmoment/1 -> Divide/1
  [dT] -> Product2/2, Product1/2, Math Function/1
  Divide/1 -> Gain/1, Product2/1  "dOm/dt"
  Sum2/1 -> Memory5/1, Memory1/1, Product1/1  "Omega"
  Memory5/1 -> Sum2/1
  Product2/1 -> Sum2/2
  Sum6/1 -> Memory2/1, Azimut/1, Gain4/1  "Azimut"
  Memory2/1 -> Sum6/1
  Gain/1 -> Product3/2
  Math Function/1 -> Product3/1
  Product1/1 -> Sum7/1
  Product3/1 -> Sum7/2
  Sum7/1 -> Sum6/2
  Memory1/1 -> Omega/1, Omega1/1  "Omega"
  [m] -> Product4/3
  Math Function5/1 -> Product4/2
  Product4/1 -> Sum of Elements/1
  [nBl] -> Product4/1
  [r_eff] -> Math Function5/1
  Sum of Elements/1 -> Sum1/2
  Generatorträgheitsmoment/1 -> Sum1/1
  Triebstrangträgheitsmoment/1 -> Sum1/3
  Sum1/1 -> Trägheitsmoment/1, Divide/2
  Gain4/1 -> Azimut1/1  "Azimut"

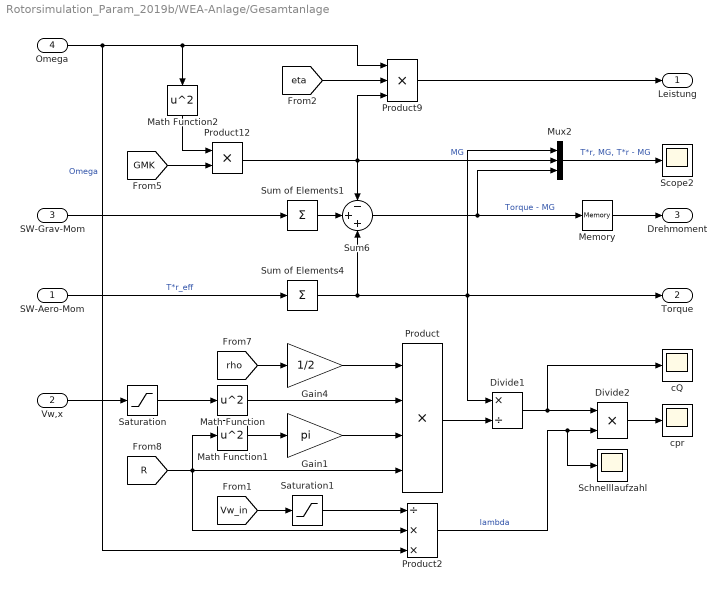
== system Rotorsimulation_Param_2019b/WEA-Anlage/Gesamtanlage ==
  SW-Aero-Mom : Inport
  Vw,x : Inport  Port=2
  SW-Grav-Mom : Inport  Port=3
  Omega : Inport  Port=4
  Divide1 : Product  Inputs=*/
  Divide2 : Product
  Gain1 : Gain  Gain=pi
  Gain4 : Gain  Gain=1/2
  Math Function : Math  Operator=square  SaturateOnIntegerOverflow=on
  Math Function1 : Math  Operator=square  SaturateOnIntegerOverflow=on
  Math Function2 : Math  Operator=square  SaturateOnIntegerOverflow=on
  Memory : Memory
  Mux2 : Mux  Inputs=3
  Product : Product  Inputs=4  RndMeth=Zero
  Product12 : Product  RndMeth=Zero
  Product2 : Product  Inputs=/**  RndMeth=Zero
  Product9 : Product  Inputs=3  RndMeth=Zero
  Saturation : Saturate  UpperLimit=inf  LowerLimit=0.1
  Saturation1 : Saturate  UpperLimit=inf  LowerLimit=0.1
  Schnelllaufzahl : Scope
  Scope2 : Scope
  Sum of Elements1 : Sum  Inputs=+
  Sum of Elements4 : Sum  Inputs=+
  Sum6 : Sum  Inputs=-++
  cQ : Scope
  cpr : Scope
  Leistung : Outport  VectorParamsAs1DForOutWhenUnconnected=off
  Torque : Outport  Port=2  VectorParamsAs1DForOutWhenUnconnected=off
  Drehmoment : Outport  Port=3  VectorParamsAs1DForOutWhenUnconnected=off
  wires:
  Product2/1 -> Divide2/2, Schnelllaufzahl/1  "lambda"
  Divide2/1 -> cpr/1
  Math Function/1 -> Product/2
  [R] -> Math Function1/1, Product/4, Product2/2
  Math Function1/1 -> Gain1/1
  Gain4/1 -> Product/1
  Gain1/1 -> Product/3
  Product/1 -> Divide1/2
  Divide1/1 -> Divide2/1, cQ/1
  Sum of Elements4/1 -> Sum6/3, Divide1/1, Mux2/1, Torque/1
  Vw,x/1 -> Saturation/1
  [rho] -> Gain4/1
  Saturation/1 -> Math Function/1
  Mux2/1 -> Scope2/1  "T*r, MG, T*r - MG"
  Sum6/1 -> Mux2/3, Memory/1  "Torque - MG"
  SW-Grav-Mom/1 -> Sum of Elements1/1
  [eta] -> Product9/2
  Product12/1 -> Product9/3, Sum6/1, Mux2/2  "MG"
  Omega/1 -> Math Function2/1, Product9/1, Product2/3  "Omega"
  [GMK] -> Product12/2
  Product9/1 -> Leistung/1
  Math Function2/1 -> Product12/1
  SW-Aero-Mom/1 -> Sum of Elements4/1  "T*r_eff"
  [Vw_in] -> Saturation1/1
  Saturation1/1 -> Product2/1
  Sum of Elements1/1 -> Sum6/2
  Memory/1 -> Drehmoment/1

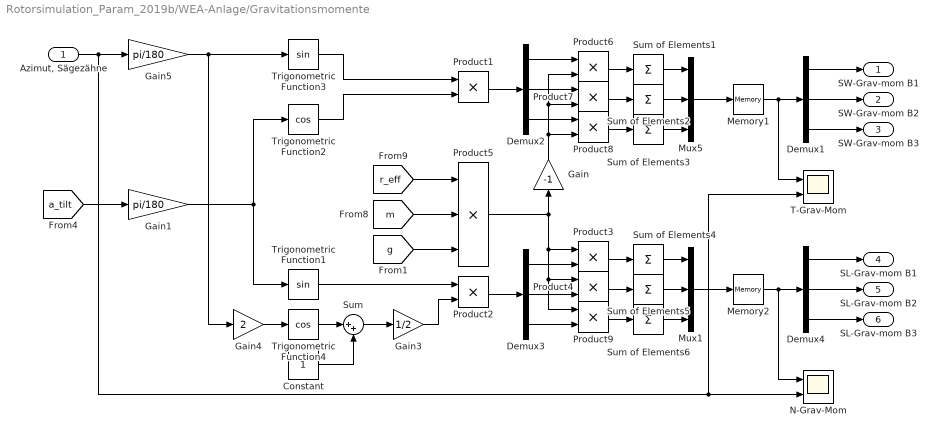
== system Rotorsimulation_Param_2019b/WEA-Anlage/Gravitationsmomente ==
  "Azimut, Sägezähne" : Inport
  Constant : Constant
  Demux{1..4} (4 alike) : Demux  Outputs=3
  Gain : Gain  Gain=-1
  Gain1 : Gain  Gain=pi/180
  Gain3 : Gain  Gain=1/2
  Gain4 : Gain  Gain=2
  Gain5 : Gain  Gain=pi/180
  Memory1 : Memory
  Memory2 : Memory
  Mux1 : Mux  Inputs=3
  Mux5 : Mux  Inputs=3
  N-Grav-Mom : Scope  NumInputPorts=2
  Product{1..4,6..9} (8 alike) : Product  RndMeth=Zero
  Product5 : Product  Inputs=3  RndMeth=Zero
  Sum : Sum  Inputs=|++
  Sum of Elements{1..6} (6 alike) : Sum  Inputs=+
  T-Grav-Mom : Scope  NumInputPorts=2
  Trigonometric Function1 : Trigonometry
  Trigonometric Function2 : Trigonometry  Operator=cos
  Trigonometric Function3 : Trigonometry
  Trigonometric Function4 : Trigonometry  Operator=cos
  SW-Grav-mom B1 : Outport  VectorParamsAs1DForOutWhenUnconnected=off
  SW-Grav-mom B2 : Outport  Port=2  VectorParamsAs1DForOutWhenUnconnected=off
  SW-Grav-mom B3 : Outport  Port=3  VectorParamsAs1DForOutWhenUnconnected=off
  SL-Grav-mom B1 : Outport  Port=4  VectorParamsAs1DForOutWhenUnconnected=off
  SL-Grav-mom B2 : Outport  Port=5  VectorParamsAs1DForOutWhenUnconnected=off
  SL-Grav-mom B3 : Outport  Port=6  VectorParamsAs1DForOutWhenUnconnected=off
  wires:
  Gain5/1 -> Trigonometric Function3/1, Gain4/1
  Product5/1 -> Gain/1, Product3/1, Product4/1, Product9/1
  "Azimut, Sägezähne"/1 -> Gain5/1, N-Grav-Mom/2, T-Grav-Mom/2
  Memory1/1 -> Demux1/1, T-Grav-Mom/1
  Product6/1 -> Sum of Elements1/1
  Sum of Elements1/1 -> Mux5/1
  Product7/1 -> Sum of Elements2/1
  Product8/1 -> Sum of Elements3/1
  Sum of Elements2/1 -> Mux5/2
  Sum of Elements3/1 -> Mux5/3
  Demux2/1 -> Product6/1
  Demux2/2 -> Product7/1
  Demux2/3 -> Product8/1
  Mux5/1 -> Memory1/1
  [r_eff] -> Product5/1
  [m] -> Product5/2
  Demux1/1 -> SW-Grav-mom B1/1
  Demux1/2 -> SW-Grav-mom B2/1
  Demux1/3 -> SW-Grav-mom B3/1
  [g] -> Product5/3
  Gain/1 -> Product6/2, Product7/2, Product8/2
  Trigonometric Function4/1 -> Sum/1
  Sum/1 -> Gain3/1
  Constant/1 -> Sum/2
  Gain3/1 -> Product2/2
  [a_tilt] -> Gain1/1
  Gain1/1 -> Trigonometric Function2/1, Trigonometric Function1/1
  Trigonometric Function3/1 -> Product1/1
  Trigonometric Function2/1 -> Product1/2
  Product1/1 -> Demux2/1
  Gain4/1 -> Trigonometric Function4/1
  Trigonometric Function1/1 -> Product2/1
  Product2/1 -> Demux3/1
  Memory2/1 -> Demux4/1, N-Grav-Mom/1
  Product3/1 -> Sum of Elements4/1
  Sum of Elements4/1 -> Mux1/1
  Product4/1 -> Sum of Elements5/1
  Product9/1 -> Sum of Elements6/1
  Sum of Elements5/1 -> Mux1/2
  Sum of Elements6/1 -> Mux1/3
  Mux1/1 -> Memory2/1
  Demux4/1 -> SL-Grav-mom B1/1
  Demux4/2 -> SL-Grav-mom B2/1
  Demux4/3 -> SL-Grav-mom B3/1
  Demux3/3 -> Product9/2
  Demux3/2 -> Product4/2
  Demux3/1 -> Product3/2

== system Rotorsimulation_Param_2019b/WEA-Anlage/Sägezähne ==
  Azimut : Inport
  Add4 : Sum
  Add5 : Sum
  Azimute : Scope
  Gain4 : Gain  Gain=180/pi
  Gain6 : Gain  Gain=2
  Generator- moment1 : Constant  Value=-120
  Grad : Constant  Value=0
  Grad1 : Constant  Value=360
  Memory1 : Memory
  Memory2 : Memory
  Memory4 : Memory
  Mux4 : Mux  Inputs=3
  Sum2 : Sum  Inputs=|+-
  Sum3 : Sum  Inputs=|++
  Sum4 : Sum  Inputs=+|+
  Sum5 : Sum  Inputs=|+-
  Switch : Switch  Threshold=360
  Sägezähne : Outport  VectorParamsAs1DForOutWhenUnconnected=off
  wires:
  Grad/1 -> Switch/3
  Grad1/1 -> Switch/1
  Gain4/1 -> Sum2/1, Sum5/1, Memory4/1  "Azimut"
  Switch/1 -> Sum3/1
  Sum2/1 -> Memory1/1, Mux4/1, Add4/1, Add5/1  "Azimut"
  Sum3/1 -> Memory2/1, Sum2/2  "Omega"
  Memory2/1 -> Sum3/2
  Sum4/1 -> Switch/2
  Sum5/1 -> Sum4/2
  Memory4/1 -> Sum5/2
  Azimut/1 -> Gain4/1
  Memory1/1 -> Sum4/1
  Generator- moment1/1 -> Add4/2, Gain6/1
  Add4/1 -> Mux4/2
  Mux4/1 -> Sägezähne/1, Azimute/1  "Azimut"
  Add5/1 -> Mux4/3
  Gain6/1 -> Add5/2

== system Rotorsimulation_Param_2019b/Drehzahl-Regler/PI-Regler/Diskreter Integrierer ==
  In1 : Inport
  0.1 : Gain  Gain=0.1
  BodyDelay2 : Delay  DelayLength=1
  BodyLSum1 : Sum  Inputs=|++  RndMeth=Nearest  SaturateOnIntegerOverflow=on  OutDataTypeStr=Inherit: Same as first input
  Product2 : Product  RndMeth=Zero
  Out1 : Outport  VectorParamsAs1DForOutWhenUnconnected=off
  wires:
  [dT] -> 0.1/1
  BodyLSum1/1 -> BodyDelay2/1
  BodyDelay2/1 -> Product2/1, BodyLSum1/2
  0.1/1 -> Product2/2
  In1/1 -> BodyLSum1/1
  Product2/1 -> Out1/1

== system Rotorsimulation_Param_2019b/WEA-Anlage/Abwindmodelle/vi-global ==
  Abs : Abs
  B1 : Constant  Value=100
  Divide : Product  Inputs=**/
  Divide1 : Product  Inputs=*/
  Divide2 : Product  Inputs=/*
  Divide3 : Product
  Gain : Gain  Gain=2
  Gain1 : Gain  Gain=pi
  Math Function : Math  Operator=square  SaturateOnIntegerOverflow=on
  Math Function1 : Math  Operator=sqrt  SaturateOnIntegerOverflow=on
  Math Function2 : Math  Operator=square  SaturateOnIntegerOverflow=on
  Math Function3 : Math  Operator=square  SaturateOnIntegerOverflow=on
  Memory5 : Memory
  Product : Product  Inputs=3  RndMeth=Zero
  Sign : Signum
  Sum : Sum  Inputs=|++
  Sum of Elements : Sum  Inputs=+
  Sum1 : Sum  Inputs=|+-
  Sum2 : Sum  Inputs=|+-
  ra/R : Constant  Value=0.1
  viG : Outport  VectorParamsAs1DForOutWhenUnconnected=off
  wires:
  Gain/1 -> Product/1
  Math Function/1 -> Gain1/1
  Gain1/1 -> Product/2
  Product/1 -> Divide/3
  Divide/1 -> Abs/1, Sign/1
  Sum of Elements/1 -> Divide/1
  [B] -> Sum2/2, Divide1/1
  B1/1 -> Divide1/2, Sum2/1, Divide2/1
  Divide1/1 -> Sum/1
  Sum/1 -> Math Function2/1
  Math Function2/1 -> Sum1/2
  Divide2/1 -> Math Function3/1
  Math Function3/1 -> Sum1/1
  Sum1/1 -> Product/3
  [nBl] -> Divide/2
  [N] -> Sum of Elements/1
  [rho] -> Gain/1
  [R] -> Math Function/1
  ra/R/1 -> Sum/2
  Sum2/1 -> Divide2/2
  Memory5/1 -> viG/1
  Abs/1 -> Math Function1/1
  Math Function1/1 -> Divide3/1
  Sign/1 -> Divide3/2
  Divide3/1 -> Memory5/1

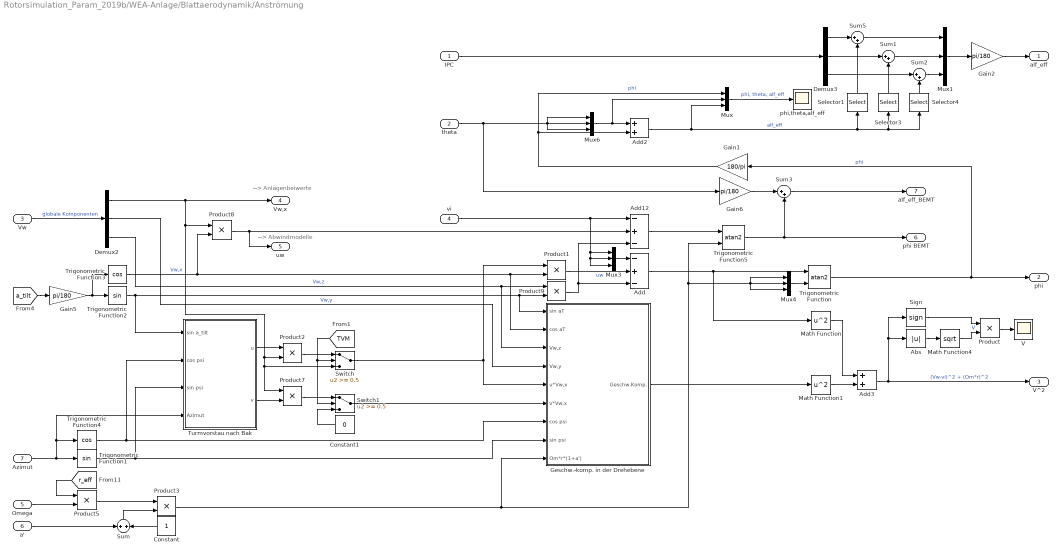
== system Rotorsimulation_Param_2019b/WEA-Anlage/Blattaerodynamik/Anströmung ==
  note: --> Abwindmodelle
  note: --> Anlagenbeiwerte
  IPC : Inport
  theta : Inport  Port=2
  Vw : Inport  Port=3
  vi : Inport  Port=4
  Omega : Inport  Port=5
  a' : Inport  Port=6
  Azimut : Inport  Port=7
  Abs : Abs
  Add : Sum  Inputs=-+-
  Add12 : Sum  Inputs=-+-
  Add2 : Sum
  Add3 : Sum
  Constant : Constant
  Constant1 : Constant  Value=0
  Demux2 : Demux  Outputs=3
  Demux3 : Demux  Outputs=3
  Gain1 : Gain  Gain=180/pi
  Gain2 : Gain  Gain=pi/180
  Gain5 : Gain  Gain=pi/180
  Gain6 : Gain  Gain=pi/180
  Geschw.-komp. in der Drehebene : Subsystem
  Math Function : Math  Operator=square  SaturateOnIntegerOverflow=on
  Math Function1 : Math  Operator=square  SaturateOnIntegerOverflow=on
  Math Function4 : Math  Operator=sqrt  SaturateOnIntegerOverflow=on
  Mux{,1,3..4,6} (5 alike) : Mux  Inputs=3
  Product{,1..3,5,7..9} (8 alike) : Product  RndMeth=Zero
  Selector1 : Selector  InputPortWidth=3*nR  IndexOptions=Index vector (dialog)  Indices=[1:nR]  OutputSizes=1
  Selector3 : Selector  InputPortWidth=3*nR  IndexOptions=Index vector (dialog)  Indices=[nR+1:2*nR]  OutputSizes=1
  Selector4 : Selector  InputPortWidth=3*nR  IndexOptions=Index vector (dialog)  Indices=[2*nR+1:3*nR]  OutputSizes=1
  Sign : Signum
  Sum : Sum  Inputs=+|+
  Sum{1..3,5} (4 alike) : Sum  Inputs=|++
  Switch : Switch  Threshold=0.5
  Switch1 : Switch  Threshold=0.5
  Trigonometric Function : Trigonometry  Operator=atan2
  Trigonometric Function1 : Trigonometry
  Trigonometric Function2 : Trigonometry
  Trigonometric Function3 : Trigonometry  Operator=cos
  Trigonometric Function4 : Trigonometry  Operator=cos
  Trigonometric Function5 : Trigonometry  Operator=atan2
  Turmvorstau nach Bak : Subsystem
  V : Scope
  phi,theta,alf_eff : Scope
  alf_eff : Outport  VectorParamsAs1DForOutWhenUnconnected=off
  phi : Outport  Port=2  VectorParamsAs1DForOutWhenUnconnected=off
  V^2 : Outport  Port=3  VectorParamsAs1DForOutWhenUnconnected=off
  Vw,x : Outport  Port=4  VectorParamsAs1DForOutWhenUnconnected=off
  uw : Outport  Port=5  VectorParamsAs1DForOutWhenUnconnected=off
  phi BEMT : Outport  Port=6  VectorParamsAs1DForOutWhenUnconnected=off
  alf_eff_BEMT : Outport  Port=7  VectorParamsAs1DForOutWhenUnconnected=off
  wires:
  Trigonometric Function/1 -> Gain1/1, phi/1  "phi"
  Mux/1 -> phi,theta,alf_eff/1  "phi, theta, alf_eff"
  Gain1/1 -> Mux/1, Add2/2  "phi"
  Gain2/1 -> alf_eff/1
  Math Function1/1 -> Add3/2
  Math Function/1 -> Add3/1
  Add3/1 -> V^2/1, Abs/1, Sign/1  "(Vw-vi)^2 + (Om*r)^2"
  Math Function4/1 -> Product/2  "V"
  Add/1 -> Trigonometric Function/1, Math Function/1
  Omega/1 -> Product5/2
  [r_eff] -> Product5/1
  Mux3/1 -> Add/1
  Sum/1 -> Product3/2
  IPC/1 -> Demux3/1
  Abs/1 -> Math Function4/1
  Sign/1 -> Product/1
  Product/1 -> V/1
  Azimut/1 -> Trigonometric Function1/1, Trigonometric Function4/1, Turmvorstau nach Bak/4(Azimut)
  Trigonometric Function1/1 -> Turmvorstau nach Bak/3(sin psi), Geschw.-komp. in der Drehebene/8(sin psi)
  Product5/1 -> Product3/1
  [a_tilt] -> Gain5/1
  Trigonometric Function2/1 -> Product9/2, Geschw.-komp. in der Drehebene/1(sin aT), Turmvorstau nach Bak/1(sin a_tilt)
  Gain5/1 -> Trigonometric Function2/1, Trigonometric Function3/1
  Trigonometric Function3/1 -> Product8/2, Product1/2, Geschw.-komp. in der Drehebene/2(cos aT)
  Product1/1 -> Add/2  "uw"
  Demux2/1 -> Vw,x/1, Product8/1, Product2/2, Product7/1, Switch/3  "Vw,x"
  Demux2/3 -> Product9/1, Geschw.-komp. in der Drehebene/3(Vw,z)  "Vw,z"
  Product9/1 -> Add/3, Add12/3
  Geschw.-komp. in der Drehebene/1(Geschw.Komp.) -> Math Function1/1
  Trigonometric Function4/1 -> Turmvorstau nach Bak/2(cos psi), Geschw.-komp. in der Drehebene/7(cos psi)
  Vw/1 -> Demux2/1  "globale Komponenten"
  Demux2/2 -> Geschw.-komp. in der Drehebene/4(Vw,y)  "Vw,y"
  Product3/1 -> Mux4/1, Mux4/2, Mux4/3, Trigonometric Function5/2, Geschw.-komp. in der Drehebene/9(Om*r*(1+a'))
  Turmvorstau nach Bak/1(u) -> Product2/1
  Turmvorstau nach Bak/2(v) -> Product7/2
  Product8/1 -> uw/1, Add12/2
  Switch/1 -> Product1/1, Geschw.-komp. in der Drehebene/5(u*Vw,x)
  vi/1 -> Add12/1, Mux3/1, Mux3/2, Mux3/3
  [TVM] -> Switch/2, Switch1/2
  Product2/1 -> Switch/1
  Product7/1 -> Switch1/1
  Constant1/1 -> Switch1/3
  Mux4/1 -> Trigonometric Function/2
  theta/1 -> Mux6/3, Mux6/1, Mux6/2, Gain6/1
  Mux6/1 -> Add2/1, Mux/2
  Add2/1 -> Mux/3, Selector1/1, Selector3/1, Selector4/1  "alf_eff"
  Mux1/1 -> Gain2/1
  Selector1/1 -> Sum5/2
  Demux3/1 -> Sum5/1
  Sum5/1 -> Mux1/1
  Selector3/1 -> Sum1/2
  Selector4/1 -> Sum2/2
  Sum2/1 -> Mux1/3
  Demux3/3 -> Sum2/1
  Sum1/1 -> Mux1/2
  Demux3/2 -> Sum1/1
  Add12/1 -> Trigonometric Function5/1
  Trigonometric Function5/1 -> phi BEMT/1, Sum3/2
  Sum3/1 -> alf_eff_BEMT/1
  Switch1/1 -> Geschw.-komp. in der Drehebene/6(v*Vw,x)
  a'/1 -> Sum/1
  Constant/1 -> Sum/2
  Gain6/1 -> Sum3/1

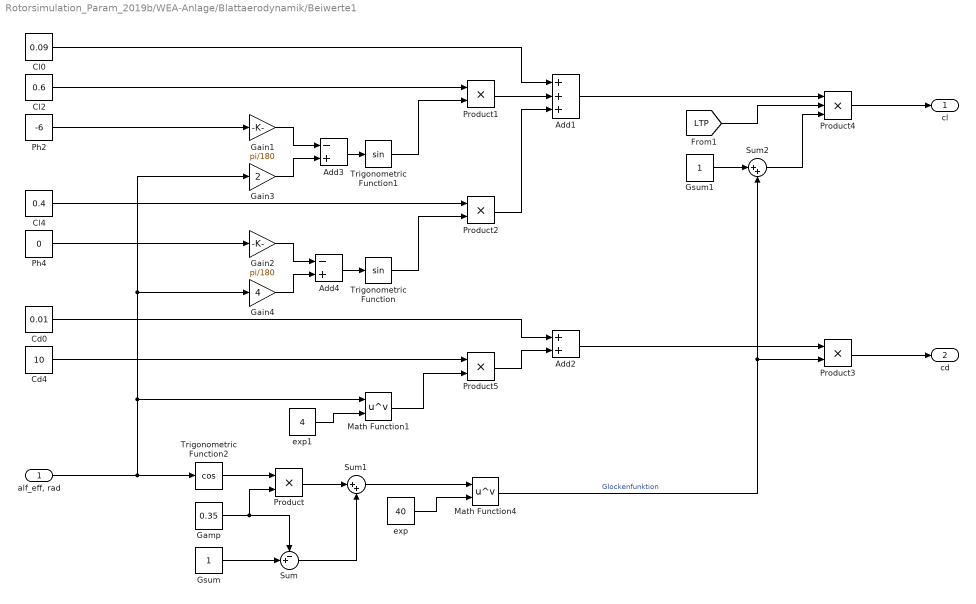
== system Rotorsimulation_Param_2019b/WEA-Anlage/Blattaerodynamik/Beiwerte1 ==
  "alf_eff, rad" : Inport
  Add1 : Sum  Inputs=+++
  Add2 : Sum
  Add3 : Sum  Inputs=-+
  Add4 : Sum  Inputs=-+
  Cd0 : Constant  Value=0.01
  Cd4 : Constant  Value=10
  Cl0 : Constant  Value=0.09
  Cl2 : Constant  Value=0.6
  Cl4 : Constant  Value=0.4
  Gain1 : Gain  Gain=pi/180
  Gain2 : Gain  Gain=pi/180
  Gain3 : Gain  Gain=2
  Gain4 : Gain  Gain=4
  Gamp : Constant  Value=0.35
  Gsum : Constant
  Gsum1 : Constant
  Math Function1 : Math  Operator=pow  SaturateOnIntegerOverflow=on
  Math Function4 : Math  Operator=pow  SaturateOnIntegerOverflow=on
  Ph2 : Constant  Value=-6
  Ph4 : Constant  Value=0
  Product{,1..3,5} (5 alike) : Product  RndMeth=Zero
  Product4 : Product  Inputs=3  RndMeth=Zero
  Sum : Sum  Inputs=-+|
  Sum1 : Sum  Inputs=|++
  Sum2 : Sum  Inputs=|++
  Trigonometric Function : Trigonometry
  Trigonometric Function1 : Trigonometry
  Trigonometric Function2 : Trigonometry  Operator=cos
  exp : Constant  Value=40
  exp1 : Constant  Value=4
  cl : Outport  VectorParamsAs1DForOutWhenUnconnected=off
  cd : Outport  Port=2  VectorParamsAs1DForOutWhenUnconnected=off
  wires:
  [LTP] -> Product4/2
  Add2/1 -> Product3/1
  Product3/1 -> cd/1
  "alf_eff, rad"/1 -> Gain3/1, Gain4/1, Math Function1/1, Trigonometric Function2/1
  Product4/1 -> cl/1
  Add1/1 -> Product4/1
  Sum2/1 -> Product4/3
  Gsum1/1 -> Sum2/1
  Math Function4/1 -> Product3/2, Sum2/2  "Glockenfunktion"
  Sum1/1 -> Math Function4/1
  Product/1 -> Sum1/1
  Sum/1 -> Sum1/2
  Trigonometric Function2/1 -> Product/1
  Gamp/1 -> Product/2, Sum/1
  Gsum/1 -> Sum/2
  Product2/1 -> Add1/3
  Trigonometric Function/1 -> Product2/2
  Cl4/1 -> Product2/1
  Gain4/1 -> Add4/2
  Gain2/1 -> Add4/1
  Add4/1 -> Trigonometric Function/1
  Trigonometric Function1/1 -> Product1/2
  Cl2/1 -> Product1/1
  Add3/1 -> Trigonometric Function1/1
  Gain3/1 -> Add3/2
  Gain1/1 -> Add3/1
  Ph4/1 -> Gain2/1
  Ph2/1 -> Gain1/1
  Cl0/1 -> Add1/1
  Product1/1 -> Add1/2
  Cd0/1 -> Add2/1
  Cd4/1 -> Product5/1
  Product5/1 -> Add2/2
  Math Function1/1 -> Product5/2
  exp/1 -> Math Function4/2
  exp1/1 -> Math Function1/2

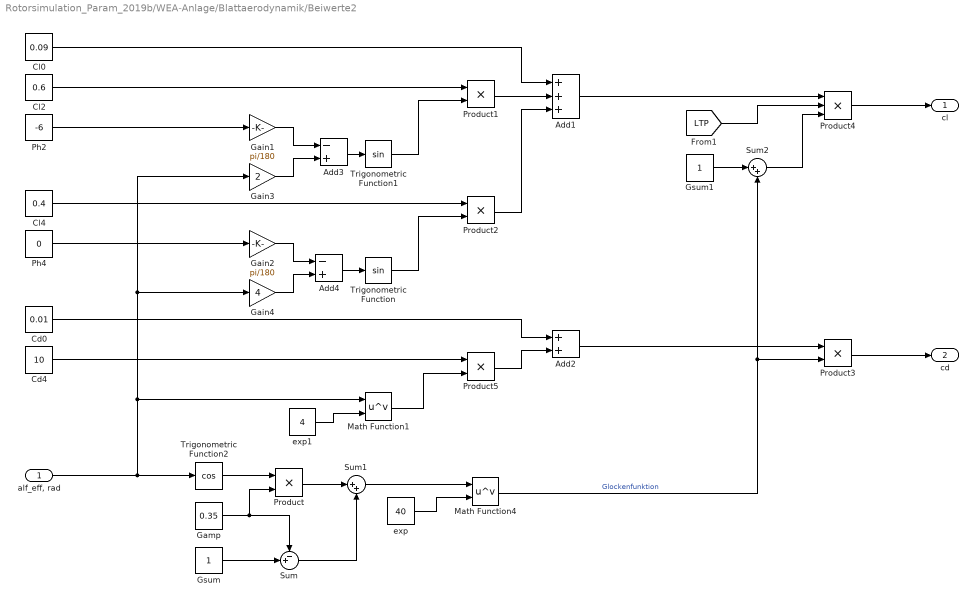
== system Rotorsimulation_Param_2019b/WEA-Anlage/Blattaerodynamik/Beiwerte2 ==
  "alf_eff, rad" : Inport
  Add1 : Sum  Inputs=+++
  Add2 : Sum
  Add3 : Sum  Inputs=-+
  Add4 : Sum  Inputs=-+
  Cd0 : Constant  Value=0.01
  Cd4 : Constant  Value=10
  Cl0 : Constant  Value=0.09
  Cl2 : Constant  Value=0.6
  Cl4 : Constant  Value=0.4
  Gain1 : Gain  Gain=pi/180
  Gain2 : Gain  Gain=pi/180
  Gain3 : Gain  Gain=2
  Gain4 : Gain  Gain=4
  Gamp : Constant  Value=0.35
  Gsum : Constant
  Gsum1 : Constant
  Math Function1 : Math  Operator=pow  SaturateOnIntegerOverflow=on
  Math Function4 : Math  Operator=pow  SaturateOnIntegerOverflow=on
  Ph2 : Constant  Value=-6
  Ph4 : Constant  Value=0
  Product{,1..3,5} (5 alike) : Product  RndMeth=Zero
  Product4 : Product  Inputs=3  RndMeth=Zero
  Sum : Sum  Inputs=-+|
  Sum1 : Sum  Inputs=|++
  Sum2 : Sum  Inputs=|++
  Trigonometric Function : Trigonometry
  Trigonometric Function1 : Trigonometry
  Trigonometric Function2 : Trigonometry  Operator=cos
  exp : Constant  Value=40
  exp1 : Constant  Value=4
  cl : Outport  VectorParamsAs1DForOutWhenUnconnected=off
  cd : Outport  Port=2  VectorParamsAs1DForOutWhenUnconnected=off
  wires:
  exp1/1 -> Math Function1/2
  exp/1 -> Math Function4/2
  Math Function1/1 -> Product5/2
  Product5/1 -> Add2/2
  Cd4/1 -> Product5/1
  Cd0/1 -> Add2/1
  Product1/1 -> Add1/2
  Cl0/1 -> Add1/1
  Ph2/1 -> Gain1/1
  Ph4/1 -> Gain2/1
  Gain1/1 -> Add3/1
  Gain3/1 -> Add3/2
  Add3/1 -> Trigonometric Function1/1
  Cl2/1 -> Product1/1
  Trigonometric Function1/1 -> Product1/2
  Add4/1 -> Trigonometric Function/1
  Gain2/1 -> Add4/1
  Gain4/1 -> Add4/2
  Cl4/1 -> Product2/1
  Trigonometric Function/1 -> Product2/2
  Product2/1 -> Add1/3
  Gsum/1 -> Sum/2
  Gamp/1 -> Sum/1, Product/2
  Trigonometric Function2/1 -> Product/1
  Sum/1 -> Sum1/2
  Product/1 -> Sum1/1
  Sum1/1 -> Math Function4/1
  Math Function4/1 -> Sum2/2, Product3/2  "Glockenfunktion"
  Gsum1/1 -> Sum2/1
  Sum2/1 -> Product4/3
  Add1/1 -> Product4/1
  Product4/1 -> cl/1
  "alf_eff, rad"/1 -> Trigonometric Function2/1, Math Function1/1, Gain4/1, Gain3/1
  Product3/1 -> cd/1
  Add2/1 -> Product3/1
  [LTP] -> Product4/2

== system Rotorsimulation_Param_2019b/WEA-Anlage/Blattaerodynamik/Blattbiegemomente ==
  T : Inport
  N : Inport  Port=2
  Demux : Demux  Outputs=3
  Demux1 : Demux  Outputs=3
  Mux1 : Mux  Inputs=3
  Mux5 : Mux  Inputs=3
  Product{1..6} (6 alike) : Product  RndMeth=Zero
  Sum of Elements{1..6} (6 alike) : Sum  Inputs=+
  SW-Aero-Mom : Outport  VectorParamsAs1DForOutWhenUnconnected=off
  SL-Aero-Mom : Outport  Port=2  VectorParamsAs1DForOutWhenUnconnected=off
  wires:
  Demux/1 -> Product1/1
  Demux/3 -> Product3/1
  Demux/2 -> Product2/1
  Product3/1 -> Sum of Elements2/1
  Product2/1 -> Sum of Elements1/1
  Product1/1 -> Sum of Elements4/1
  Sum of Elements4/1 -> Mux5/1
  Sum of Elements1/1 -> Mux5/2
  Sum of Elements2/1 -> Mux5/3
  [r_eff] -> Product1/2, Product2/2, Product3/2, Product4/2, Product5/2, Product6/2
  Demux1/1 -> Product4/1
  Demux1/3 -> Product6/1
  Demux1/2 -> Product5/1
  Product6/1 -> Sum of Elements5/1
  Product5/1 -> Sum of Elements3/1
  Product4/1 -> Sum of Elements6/1
  Sum of Elements6/1 -> Mux1/1
  Sum of Elements3/1 -> Mux1/2
  Sum of Elements5/1 -> Mux1/3
  Mux5/1 -> SW-Aero-Mom/1
  Mux1/1 -> SL-Aero-Mom/1
  N/1 -> Demux1/1
  T/1 -> Demux/1

== system Rotorsimulation_Param_2019b/WEA-Anlage/Blattaerodynamik/Komponenten für BEMT ==
  "phi, BEMT" : Inport
  cl : Inport  Port=2
  cd : Inport  Port=3
  Produc1 : Product  RndMeth=Zero
  Product10 : Product  RndMeth=Zero
  Product12 : Product  RndMeth=Zero
  Product16 : Product  RndMeth=Zero
  Sum2 : Sum  Inputs=|+-
  Sum3 : Sum  Inputs=|++
  Trigonometric Function5 : Trigonometry  Operator=cos
  Trigonometric Function7 : Trigonometry
  sin phi : Outport  VectorParamsAs1DForOutWhenUnconnected=off
  cos phi : Outport  Port=2  VectorParamsAs1DForOutWhenUnconnected=off
  ct : Outport  Port=3  VectorParamsAs1DForOutWhenUnconnected=off
  cn : Outport  Port=4  VectorParamsAs1DForOutWhenUnconnected=off
  wires:
  Produc1/1 -> Sum2/2  "cos CD"
  Product16/1 -> Sum2/1  "sin CL"
  "phi, BEMT"/1 -> Trigonometric Function5/1, Trigonometric Function7/1
  Product12/1 -> Sum3/2  "sin CD"
  Product10/1 -> Sum3/1  "cos CL"
  cl/1 -> Product16/2, Product10/2
  cd/1 -> Produc1/2, Product12/2
  Sum2/1 -> ct/1  "Ct"
  Sum3/1 -> cn/1  "Cn"
  Trigonometric Function7/1 -> Product16/1, Product12/1, sin phi/1
  Trigonometric Function5/1 -> Produc1/1, Product10/1, cos phi/1
